simulink library "INP_DRVR_EB"  (R2023b)
settings: Solver=VariableStepAuto  StartTime=0.0  StopTime=10.0  RelTol=1e-3
undefined symbols (not defined in the file or in its folder): p_RatStCoef1_na, p_RatStCoef2_na
settings Model: Creator=blatak  LastModifiedBy=blatak

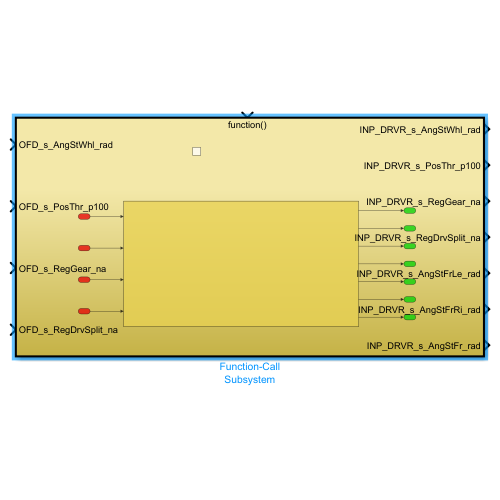
[thumbnail: Simulink's stored preview of the top-level diagram]
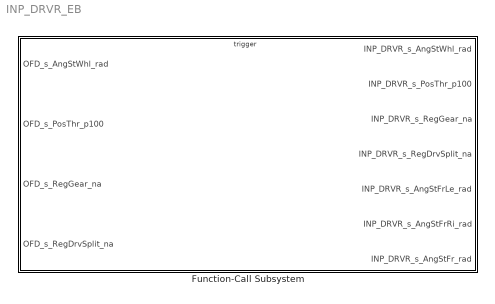
== system INP_DRVR_EB ==
  Function-Call Subsystem : Subsystem  TreatAsAtomicUnit=on

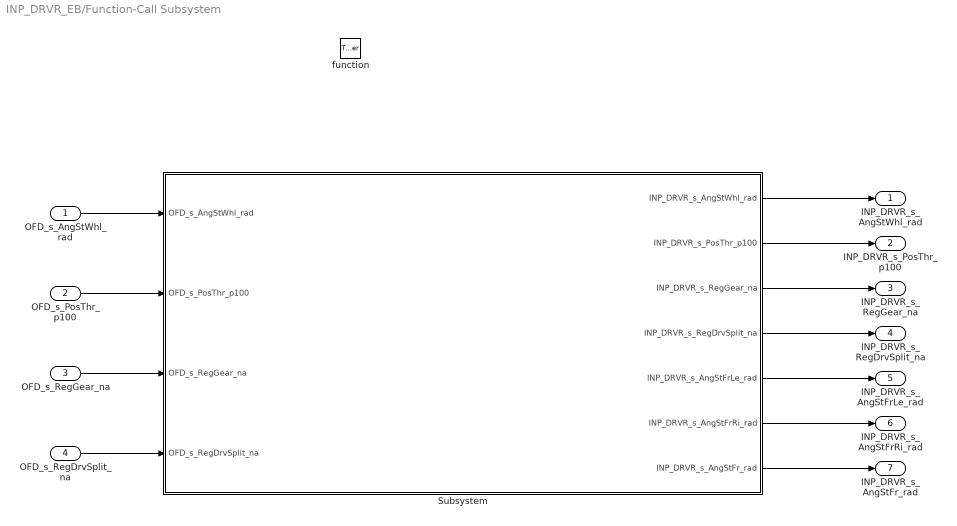
== system INP_DRVR_EB/Function-Call Subsystem ==
  OFD_s_AngStWhl_rad : Inport
  OFD_s_PosThr_p100 : Inport  Port=2
  OFD_s_RegGear_na : Inport  Port=3
  OFD_s_RegDrvSplit_na : Inport  Port=4
  function : TriggerPort  TriggerType=function-call  VariantControl=(inherit)
  Subsystem : Subsystem
  INP_DRVR_s_AngStWhl_rad : Outport
  INP_DRVR_s_PosThr_p100 : Outport  Port=2
  INP_DRVR_s_RegGear_na : Outport  Port=3
  INP_DRVR_s_RegDrvSplit_na : Outport  Port=4
  INP_DRVR_s_AngStFrLe_rad : Outport  Port=5
  INP_DRVR_s_AngStFrRi_rad : Outport  Port=6
  INP_DRVR_s_AngStFr_rad : Outport  Port=7
  wires:
  OFD_s_AngStWhl_rad/1 -> Subsystem/1(OFD_s_AngStWhl_rad)
  OFD_s_PosThr_p100/1 -> Subsystem/2(OFD_s_PosThr_p100)
  OFD_s_RegGear_na/1 -> Subsystem/3(OFD_s_RegGear_na)
  OFD_s_RegDrvSplit_na/1 -> Subsystem/4(OFD_s_RegDrvSplit_na)
  Subsystem/1(INP_DRVR_s_AngStWhl_rad) -> INP_DRVR_s_AngStWhl_rad/1
  Subsystem/2(INP_DRVR_s_PosThr_p100) -> INP_DRVR_s_PosThr_p100/1
  Subsystem/3(INP_DRVR_s_RegGear_na) -> INP_DRVR_s_RegGear_na/1
  Subsystem/4(INP_DRVR_s_RegDrvSplit_na) -> INP_DRVR_s_RegDrvSplit_na/1
  Subsystem/5(INP_DRVR_s_AngStFrLe_rad) -> INP_DRVR_s_AngStFrLe_rad/1
  Subsystem/6(INP_DRVR_s_AngStFrRi_rad) -> INP_DRVR_s_AngStFrRi_rad/1
  Subsystem/7(INP_DRVR_s_AngStFr_rad) -> INP_DRVR_s_AngStFr_rad/1

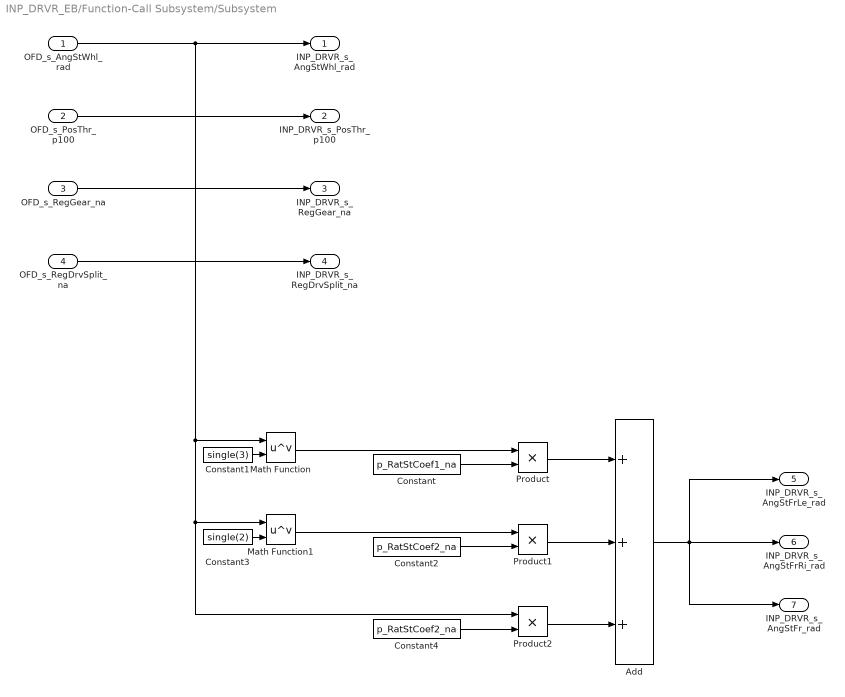
== system INP_DRVR_EB/Function-Call Subsystem/Subsystem ==
  OFD_s_AngStWhl_rad : Inport
  OFD_s_PosThr_p100 : Inport  Port=2
  OFD_s_RegGear_na : Inport  Port=3
  OFD_s_RegDrvSplit_na : Inport  Port=4
  Add : Sum  Inputs=+++
  Constant : Constant  Value=p_RatStCoef1_na
  Constant1 : Constant  Value=single(3)
  Constant2 : Constant  Value=p_RatStCoef2_na
  Constant3 : Constant  Value=single(2)
  Constant4 : Constant  Value=p_RatStCoef2_na
  Math Function : Math  Operator=pow
  Math Function1 : Math  Operator=pow
  Product : Product
  Product1 : Product
  Product2 : Product
  INP_DRVR_s_AngStWhl_rad : Outport
  INP_DRVR_s_PosThr_p100 : Outport  Port=2
  INP_DRVR_s_RegGear_na : Outport  Port=3
  INP_DRVR_s_RegDrvSplit_na : Outport  Port=4
  INP_DRVR_s_AngStFrLe_rad : Outport  Port=5
  INP_DRVR_s_AngStFrRi_rad : Outport  Port=6
  INP_DRVR_s_AngStFr_rad : Outport  Port=7
  wires:
  OFD_s_AngStWhl_rad/1 -> INP_DRVR_s_AngStWhl_rad/1, Product2/1, Math Function1/1, Math Function/1
  Math Function/1 -> Product/1
  Constant3/1 -> Math Function1/2
  Product1/1 -> Add/2
  Constant4/1 -> Product2/2
  Product2/1 -> Add/3
  Add/1 -> INP_DRVR_s_AngStFr_rad/1, INP_DRVR_s_AngStFrRi_rad/1, INP_DRVR_s_AngStFrLe_rad/1
  Constant/1 -> Product/2
  Constant1/1 -> Math Function/2
  Math Function1/1 -> Product1/1
  Product/1 -> Add/1
  OFD_s_PosThr_p100/1 -> INP_DRVR_s_PosThr_p100/1
  Constant2/1 -> Product1/2
  OFD_s_RegGear_na/1 -> INP_DRVR_s_RegGear_na/1
  OFD_s_RegDrvSplit_na/1 -> INP_DRVR_s_RegDrvSplit_na/1
